simulink model "HBridgeControlledDCMachine"  (R2016a)
settings: Solver=ode23tb  StartTime=0.0  StopTime=1  MaxStep=0.02  RelTol=1e-4
libraries: powerlib x8
settings Model: Creator=mrsmash  LastModifiedBy=mrsmash
settings DebuggingCC: MaxConsecutiveZCsMsg=none

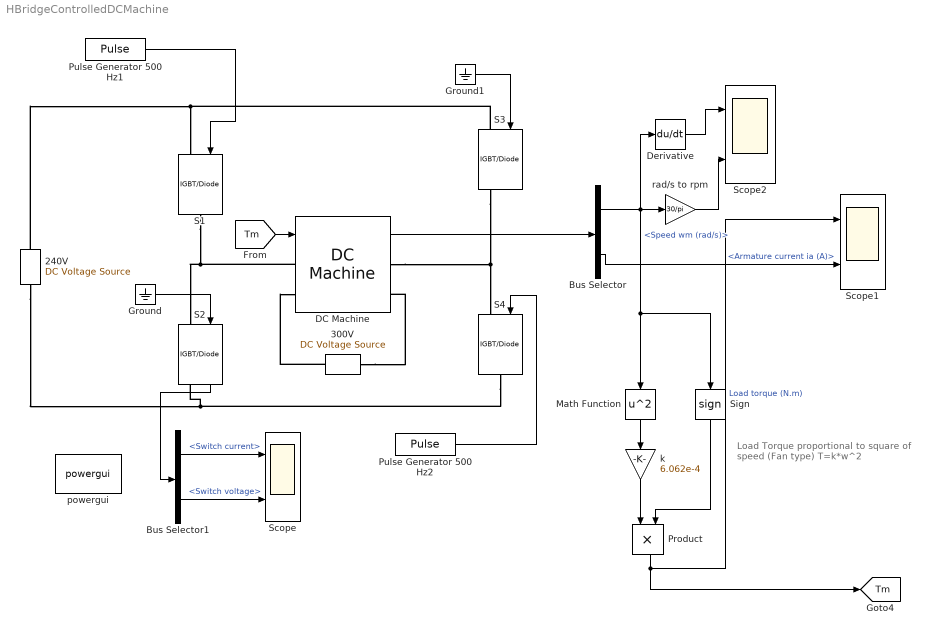
== system HBridgeControlledDCMachine ==
  note: Load Torque proportional to
      | square of speed (Fan type)
      | T=k*w^2
  240V : powerlib/Electrical Sources/DC Voltage Source  Amplitude=240  Measurements=Voltage
  300V : powerlib/Electrical Sources/DC Voltage Source  Amplitude=300  Measurements=Voltage
  Bus Selector : BusSelector  OutputSignals=Speed wm (rad/s),Armature current ia (A)
  Bus Selector1 : BusSelector  OutputSignals=Switch current,Switch voltage
  DC Machine : powerlib/Machines/DC Machine  PresetModel=01: 5HP 240V 1750RPM Field:300V  MechanicalLoad=Torque TL  FieldType=Wound  ShowDetailedParameters=on  MeasurementBus=off  RLa=[2.581 0.028]  RLf=[281.3 156]  Laf=0.9483  MachineConstant=Torque constant (N.m/A)  Ke=1.8  Kt=1.8  J=0.02215  Bm=0.002953  Tf=0.5161  w0=1  Ifinit=1  TsPowergui=0  TsBlock=-1
  Derivative : Derivative
  Ground : Ground
  Ground1 : Ground
  Math Function : Math  Operator=square  SaturateOnIntegerOverflow=on
  Product : Product  RndMeth=Zero
  Pulse Generator 500 Hz1 : DiscretePulseGenerator  PulseType=Time based  Period=2e-3  PulseWidth=75
  Pulse Generator 500 Hz2 : DiscretePulseGenerator  PulseType=Time based  Period=2e-3  PulseWidth=75
  S1 : powerlib/Power Electronics/IGBT//Diode  Ron=0.001  Rs=1e5  Cs=inf  Measurements=off
  S2 : powerlib/Power Electronics/IGBT//Diode  Ron=1e-3  Rs=1e5  Cs=inf  Measurements=on
  S3 : powerlib/Power Electronics/IGBT//Diode  Ron=1e-3  Rs=1e5  Cs=inf  Measurements=on
  S4 : powerlib/Power Electronics/IGBT//Diode  Ron=1e-3  Rs=1e5  Cs=inf  Measurements=off
  Scope : Scope  NumInputPorts=2
  Scope1 : Scope  NumInputPorts=2
  Scope2 : Scope  NumInputPorts=2
  Sign : Signum
  k : Gain  Gain=6.062e-4
  powergui : powerlib/powergui  Priority=1  SimulationMode=Continuous  SolverType=Tustin/Backward Euler (TBE)  SampleTime=50e-6  frequency=60  SPID=off  DisableSnubberDevices=off  DisableRonSwitches=off  DisableVfSwitches=off  SwTol=0  DisplayEquations=off  Interpol=off  ExternalGateDelay=off  methode=off  Ts=10  FunctionMessages=off  echomessages=off  HookPort=off  EnableUseOfTLC=off  x0status=blocks  frequencyindice=0  Pbase=100e6  ErrMax=1e-4  Iterations=50  UnitsV=kV  UnitsW=MW  buscounter=0  RestoreLinks=warning  ResistiveCurrentMeasurement=off  Frange=[0:2:500]  Ylog=off  Xlog=on  ShowGrid=off  save=off  variable=ZData  structure=0  ZoomFFT=off  StartTime=0.0  cycles=1  DisplayStyle=1  fundamental=60  FreqAxis=off  MaxFrequency=1000  frequencyindicesteady=1  RmsSteady=1  display=off
  rad/s to rpm : Gain  Gain=30/pi
  tag scope: Tm=global
  wires:
  [Tm] -> DC Machine/1
  Pulse Generator 500 Hz1/1 -> S1/1
  DC Machine/1 -> Bus Selector/1
  Bus Selector/2 -> Scope1/2  "<Armature current ia (A)>"
  Bus Selector/1 -> Derivative/1, rad/s to rpm/1, Sign/1, Math Function/1  "<Speed wm (rad/s)>"
  Math Function/1 -> k/1
  k/1 -> Product/1
  Sign/1 -> Product/2
  Product/1 -> [Tm], Scope1/1  "Load torque (N.m)"
  Pulse Generator 500 Hz2/1 -> S4/1
  Ground1/1 -> S3/1
  Ground/1 -> S2/1
  rad/s to rpm/1 -> Scope2/2
  Derivative/1 -> Scope2/1
  S2/1 -> Bus Selector1/1
  Bus Selector1/1 -> Scope/1  "<Switch current>"
  Bus Selector1/2 -> Scope/2  "<Switch voltage>"
  connections:
  S1/RConn1 -- DC Machine/LConn1 -- S2/LConn1
  S3/RConn1 -- DC Machine/RConn1 -- S4/LConn1
  240V/RConn1 -- S1/LConn1 -- S3/LConn1
  240V/LConn1 -- S2/RConn1 -- S4/RConn1
  300V/LConn1 -- DC Machine/RConn2
  300V/RConn1 -- DC Machine/LConn2
